simulink library "INT_PTCOP_TrqCnv"  (R2016b)
settings: Solver=VariableStepAuto  StartTime=0.0  StopTime=10.0  RelTol=1e-3
settings Model: Creator=yangyang  LastModifiedBy=yangyang

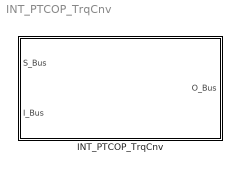
== system INT_PTCOP_TrqCnv ==
  INT_PTCOP_TrqCnv : Subsystem

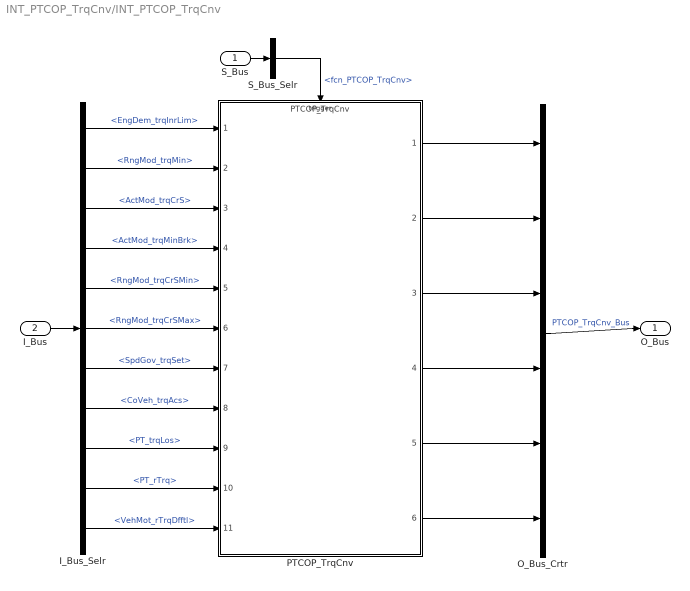
== system INT_PTCOP_TrqCnv/INT_PTCOP_TrqCnv ==
  S_Bus : Inport
  I_Bus : Inport  Port=2
  I_Bus_Selr : BusSelector  OutputSignals=EngDem_trqInrLim,RngMod_trqMin,ActMod_trqCrS,ActMod_trqMinBrk,RngMod_trqCrSMin,RngMod_trqCrSMax,SpdGov_trqSet,CoVeh_trqAcs,PT_trqLos,PT_rTrq,VehMot_rTrqDfftl
  O_Bus_Crtr : BusCreator  Inputs=6
  PTCOP_TrqCnv : ModelReference  ModelNameDialog=PTCOP_TrqCnv  SimulationMode=Normal  ModelReferenceVersion=1.5  TriggerPortName=function  TriggerPortTriggerType=function-call  TriggerPortStatesWhenEnabling=held
  S_Bus_Selr : BusSelector  OutputSignals=fcn_PTCOP_TrqCnv
  O_Bus : Outport
  wires:
  S_Bus_Selr/1 -> PTCOP_TrqCnv/Trigger  "<fcn_PTCOP_TrqCnv>"
  S_Bus/1 -> S_Bus_Selr/1
  I_Bus/1 -> I_Bus_Selr/1
  I_Bus_Selr/1 -> PTCOP_TrqCnv/1  "<EngDem_trqInrLim>"
  I_Bus_Selr/2 -> PTCOP_TrqCnv/2  "<RngMod_trqMin>"
  I_Bus_Selr/3 -> PTCOP_TrqCnv/3  "<ActMod_trqCrS>"
  I_Bus_Selr/4 -> PTCOP_TrqCnv/4  "<ActMod_trqMinBrk>"
  I_Bus_Selr/5 -> PTCOP_TrqCnv/5  "<RngMod_trqCrSMin>"
  I_Bus_Selr/6 -> PTCOP_TrqCnv/6  "<RngMod_trqCrSMax>"
  I_Bus_Selr/7 -> PTCOP_TrqCnv/7  "<SpdGov_trqSet>"
  I_Bus_Selr/8 -> PTCOP_TrqCnv/8  "<CoVeh_trqAcs>"
  I_Bus_Selr/9 -> PTCOP_TrqCnv/9  "<PT_trqLos>"
  I_Bus_Selr/10 -> PTCOP_TrqCnv/10  "<PT_rTrq>"
  I_Bus_Selr/11 -> PTCOP_TrqCnv/11  "<VehMot_rTrqDfftl>"
  O_Bus_Crtr/1 -> O_Bus/1  "PTCOP_TrqCnv_Bus"
  PTCOP_TrqCnv/1 -> O_Bus_Crtr/1
  PTCOP_TrqCnv/2 -> O_Bus_Crtr/2
  PTCOP_TrqCnv/3 -> O_Bus_Crtr/3
  PTCOP_TrqCnv/4 -> O_Bus_Crtr/4
  PTCOP_TrqCnv/5 -> O_Bus_Crtr/5
  PTCOP_TrqCnv/6 -> O_Bus_Crtr/6
